simulink library "hydroLib3utils_R2019B"  (R2019b)
settings: Solver=ode45  StartTime=0.0  StopTime=10.0  RelTol=1e-3
undefined symbols (not defined in the file): beta, d00, d01, d1, dP, dpn, dpn_P, dpn_T, I_Anteil_x, k_stosz, klin, omega, p0, P_Anteil_x, Qlam, Qn, Qn_P, s_dyn, s_reib, t_sw, V, V0, v_0, v_fr_min, v_min, x_max, x_min, xi
libraries: simulink x15, $bdroot x6, hydroLib3 x2
(part 2 of 2)

== system hydroLib3utils_R2019B/Endlagen-Stosz und Reibung/Stribeck Reibung/Subsystem1/Detect Increase1 ==
  U : Inport
  FixPt Relational Operator : RelationalOperator  Operator=>  OutDataTypeStr=uint(8)  ZeroCross=off  RndMeth=Nearest
  Memory : Memory
  Y : Outport  InitialOutput=0
  wires:
  FixPt Relational Operator/1 -> Y/1  "Edge"
  Memory/1 -> FixPt Relational Operator/2  "U(k-1)"
  U/1 -> FixPt Relational Operator/1, Memory/1  "U(k)"

== system hydroLib3utils_R2019B/Endlagen-Stosz und Reibung/Stribeck Reibung/Subsystem1/Detect Increase2 ==
  U : Inport
  FixPt Relational Operator : RelationalOperator  Operator=>  OutDataTypeStr=uint(8)  ZeroCross=off  RndMeth=Nearest
  Memory : Memory
  Y : Outport  InitialOutput=0
  wires:
  U/1 -> Memory/1, FixPt Relational Operator/1  "U(k)"
  Memory/1 -> FixPt Relational Operator/2  "U(k-1)"
  FixPt Relational Operator/1 -> Y/1  "Edge"

== matlab function hydroLib3utils_R2019B/sqrt w// approx/MATLAB Function ==
  data: dp input; y output; pt input; kQn_dpn input; a1 input; a2 input
function y = fcn(dp,pt,kQn_dpn,a1,a2)

%dp = u(1);
%pt = u(2);

if dp >= 0
  if dp > pt
    y = kQn_dpn*sqrt(dp);
  else
    y = a1*dp-a2*dp^2;
  end
else
  if dp < -pt
    y = -kQn_dpn*sqrt(-dp);
  else
    y = a1*dp+a2*dp^2;
  end
end
